simulink model "UAV_Dynamics_Autopilot_Communication"  (R2024a)
settings: Solver=ode4  StartTime=0.0  StopTime=inf  FixedStep=SampleTime  RelTol=1e-3
undefined symbols (not defined in the file): SampleTime
libraries: px4MAVLinkBridgelib x2
settings Model: Creator=The MathWorks, Inc.  LastModifiedBy=The MathWorks, Inc.
settings SolverCC: MaxZcPerStep=1
settings ModelReferenceCC: EnableRefExpFcnMdlSchedulingChecks=on
settings RTWCC: GPUComputeCapability=3.5  DLArmComputeVersion=19.05

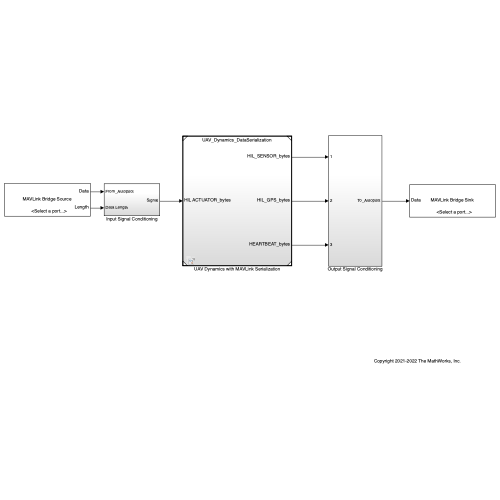
[thumbnail: Simulink's stored preview of the top-level diagram]
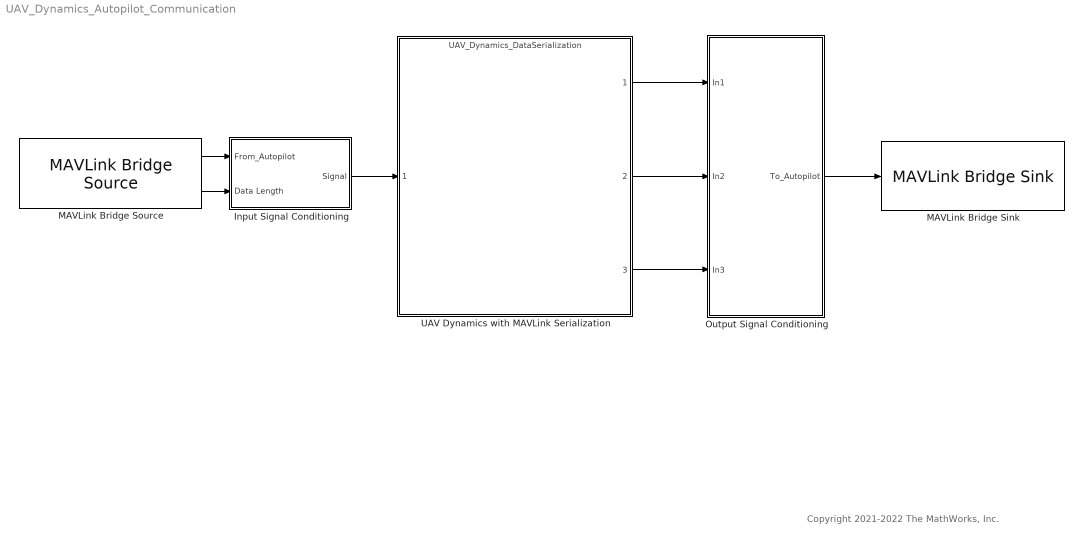
== system UAV_Dynamics_Autopilot_Communication ==
  note: Copyright 2021-2022 The MathWorks, Inc.
  Input Signal Conditioning : Subsystem
  MAVLink Bridge Sink : px4MAVLinkBridgelib/MAVLink Bridge Sink  PixhawkSerialPorttemp=Specify manually  PixhawkSerialPortManually=COM12  FieldTable={ 'UDP', '127.0.0.1', '14550' }
  MAVLink Bridge Source : px4MAVLinkBridgelib/MAVLink Bridge Source  PixhawkSerialPorttemp=Specify manually  PixhawkSerialPortManually=COM12  dataLength=MAVLink_Input_Read_Size  FieldTable={ 'UDP', '127.0.0.1', '14550' }  SampleTime=SampleTime
  Output Signal Conditioning : Subsystem
  UAV Dynamics with MAVLink Serialization : ModelReference  ModelNameDialog=UAV_Dynamics_DataSerialization.slx  SimulationMode=Normal  ModelReferenceVersion=5.0
  wires:
  UAV Dynamics with MAVLink Serialization/2 -> Output Signal Conditioning/2(In2)
  UAV Dynamics with MAVLink Serialization/1 -> Output Signal Conditioning/1(In1)
  UAV Dynamics with MAVLink Serialization/3 -> Output Signal Conditioning/3(In3)
  Input Signal Conditioning/1(Signal) -> UAV Dynamics with MAVLink Serialization/1
  MAVLink Bridge Source/1 -> Input Signal Conditioning/1(From_Autopilot)
  MAVLink Bridge Source/2 -> Input Signal Conditioning/2(Data Length)
  Output Signal Conditioning/1(To_Autopilot) -> MAVLink Bridge Sink/1

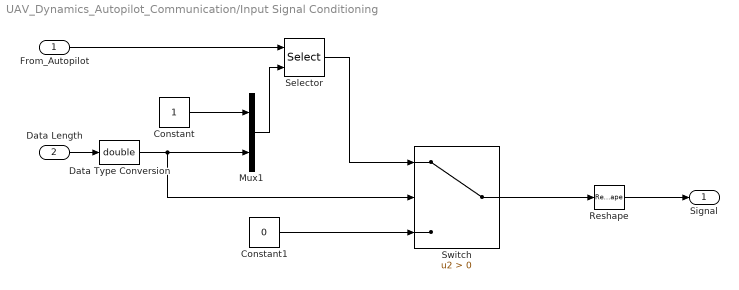
== system UAV_Dynamics_Autopilot_Communication/Input Signal Conditioning ==
  From_Autopilot : Inport
  Data Length : Inport  Port=2
  Constant : Constant
  Constant1 : Constant  Value=0  OutDataTypeStr=uint8  SampleTime=-1
  Data Type Conversion : DataTypeConversion  OutDataTypeStr=double  SaturateOnIntegerOverflow=off  RndMeth=Floor
  Mux1 : Mux  Inputs=2
  Reshape : Reshape
  Selector : Selector  InputPortWidth=MAVLink_Input_Read_Size  IndexOptions=Starting and ending indices (port)  Indices=[1 3]  OutputSizes=1
  Switch : Switch  Criteria=u2 > Threshold  SaturateOnIntegerOverflow=off  InputSameDT=off
  Signal : Outport
  wires:
  Reshape/1 -> Signal/1
  Mux1/1 -> Selector/2
  Data Length/1 -> Data Type Conversion/1
  Constant/1 -> Mux1/1
  Selector/1 -> Switch/1
  From_Autopilot/1 -> Selector/1
  Constant1/1 -> Switch/3
  Switch/1 -> Reshape/1
  Data Type Conversion/1 -> Switch/2, Mux1/2

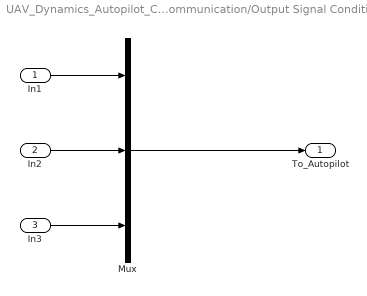
== system UAV_Dynamics_Autopilot_Communication/Output Signal Conditioning ==
  In1 : Inport
  In2 : Inport  Port=2
  In3 : Inport  Port=3
  Mux : Mux  Inputs=3
  To_Autopilot : Outport
  wires:
  Mux/1 -> To_Autopilot/1
  In2/1 -> Mux/2
  In3/1 -> Mux/3
  In1/1 -> Mux/1
